simulink model "mParametersTop"  (Simulink 8.0)
settings: Solver=FixedStepDiscrete  StartTime=0.0  StopTime=10.0  FixedStep=1  RelTol=1e-3
PostLoadFcn:
  | evalin('base','load bparams');
undefined symbols (not defined in the file or in its folder): IC_global
CloseFcn:
  | evalin('base','clear IC_global');
settings Model: FPTRunName=Active  Creator=The MathWorks Inc.  LastModifiedBy=mtocci  ExtModeAutoUpdateStatusClock=off
settings DataIOCC: SignalLoggingSaveFormat=ModelDataLogs  SignalLoggingName=logsOut
settings OptimizationCC: InlineParams=on  InlineInvariantSignals=on  InitFltsAndDblsToZero=on
settings DebuggingCC: SaveWithParameterizedLinksMsg=none  CheckExecutionContextPreStartOutputMsg=on  CheckExecutionContextRuntimeOutputMsg=on  SolverPrmCheckMsg=none  MultiTaskDSMMsg=warning  MultiTaskCondExecSysMsg=none  SigSpecEnsureSampleTimeMsg=none  FcnCallInpInsideContextMsg=Use local settings  StrictBusMsg=ErrorOnBusTreatedAsVector
settings HardwareCC: TargetHWDeviceType=32-bit Generic
settings ModelReferenceCC: UpdateModelReferenceTargets=IfOutOfDate  CheckModelReferenceTargetMessage=none
settings RTWCC: GenerateReport=on  ProcessScript=grt_make_rtw_hook  LaunchReport=on  IncludeERTFirstTime=on
settings CodeAppCC: MaxIdLength=100
settings GRTTargetCC: TargetFcnLib=ansi_tfl_tmw.mat  SharedFunctionMode=Off  CombineOutputUpdateFcns=off  GRTInterface=on

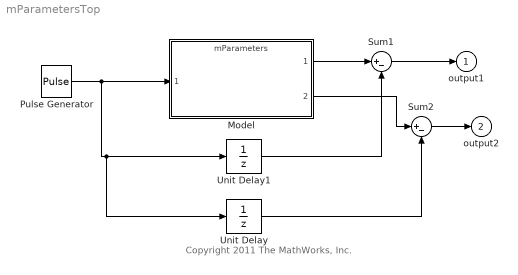
== system mParametersTop ==
  note: Copyright 2011 The MathWorks, Inc.
  Model : ModelReference  ModelNameDialog=mParameters  ParameterArgumentNames=IC_arg  ParameterArgumentValues=-5  SimulationMode=Accelerator  ModelReferenceVersion=1.84  CopyOfModelName=mParameters  DefaultDataLogging=on
  Pulse Generator : DiscretePulseGenerator
  Sum1 : Sum  Inputs=|+-
  Sum2 : Sum  Inputs=|+-
  Unit Delay : UnitDelay  X0=-5  SampleTime=-1
  Unit Delay1 : UnitDelay  X0=IC_global  SampleTime=-1
  output1 : Outport
  output2 : Outport  Port=2
  wires:
  Pulse Generator/1 -> Model/1, Unit Delay1/1, Unit Delay/1
  Model/1 -> Sum1/1
  Sum1/1 -> output1/1
  Unit Delay1/1 -> Sum1/2
  Model/2 -> Sum2/1
  Unit Delay/1 -> Sum2/2
  Sum2/1 -> output2/1
